simulink model "lab3_p7"  (R2020a)
settings: Solver=VariableStepAuto  StartTime=0.0  StopTime=stop_time  RelTol=1e-3
InitFcn:
  | sm_callback_init.m
values from neighbouring files (symbols this model uses):
  mp = sm_init_avalon_signals(mp)    [sm_callback_init.m]
settings Model: Creator=Owner  LastModifiedBy=Owner
settings DataIOCC: ReturnWorkspaceOutputs=off

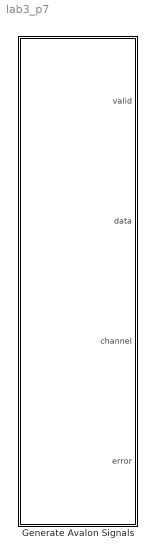
== system lab3_p7 ==
  Generate Avalon Signals : Subsystem

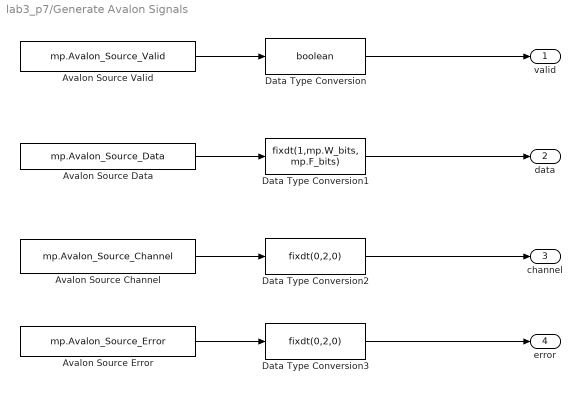
== system lab3_p7/Generate Avalon Signals ==
  Avalon Source Channel : FromWorkspace  VariableName=mp.Avalon_Source_Channel  OutDataTypeStr=double  SampleTime=mp.Ts_system
  Avalon Source Data : FromWorkspace  VariableName=mp.Avalon_Source_Data  OutDataTypeStr=double  SampleTime=mp.Ts_system
  Avalon Source Error : FromWorkspace  VariableName=mp.Avalon_Source_Error  OutDataTypeStr=double  SampleTime=mp.Ts_system
  Avalon Source Valid : FromWorkspace  VariableName=mp.Avalon_Source_Valid  OutDataTypeStr=double  SampleTime=mp.Ts_system
  Data Type Conversion : DataTypeConversion  OutDataTypeStr=boolean  RndMeth=Nearest
  Data Type Conversion1 : DataTypeConversion  OutDataTypeStr=fixdt(1,mp.W_bits, mp.F_bits)  RndMeth=Nearest
  Data Type Conversion2 : DataTypeConversion  OutDataTypeStr=fixdt(0,2,0)  RndMeth=Nearest
  Data Type Conversion3 : DataTypeConversion  OutDataTypeStr=fixdt(0,2,0)  RndMeth=Nearest
  valid : Outport
  data : Outport  Port=2
  channel : Outport  Port=3
  error : Outport  Port=4
  wires:
  Data Type Conversion/1 -> valid/1
  Avalon Source Valid/1 -> Data Type Conversion/1
  Avalon Source Data/1 -> Data Type Conversion1/1
  Data Type Conversion1/1 -> data/1
  Data Type Conversion2/1 -> channel/1
  Avalon Source Channel/1 -> Data Type Conversion2/1
  Data Type Conversion3/1 -> error/1
  Avalon Source Error/1 -> Data Type Conversion3/1
